simulink model "wheel_dynamics_model"  (R2024b)
settings: Solver=VariableStepAuto  StartTime=0.0  StopTime=3  RelTol=1e-3
undefined symbols (not defined in the file or in its folder): D1, D2, Dm, Dw, gear_ratio, J1, J2, Jm, Js1, Js2, Jw, Ks1, Ks2, tire_loaded_radius
settings Model: VariantFading=off  Creator=bglen  LastModifiedBy=37rst
settings RTWCC: GPUComputeCapability=3.5

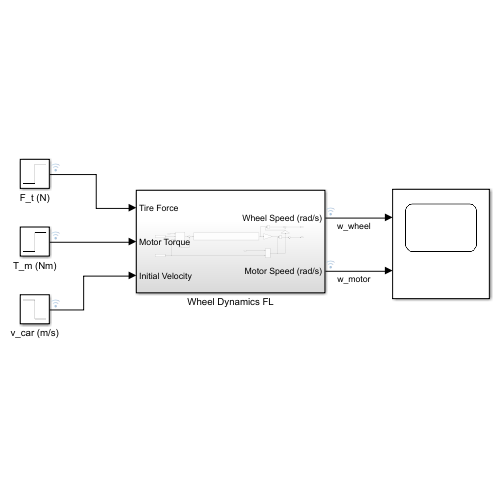
[thumbnail: Simulink's stored preview of the top-level diagram]
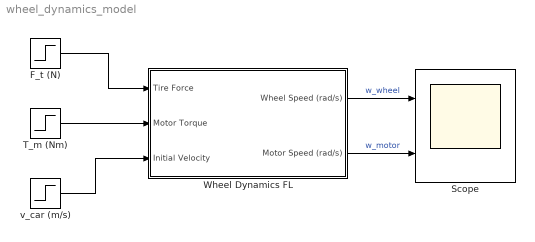
== system wheel_dynamics_model ==
  F_t (N) : Step  Time=2  After=10  SampleTime=0
  Scope : Scope  NumInputPorts=2
  T_m (Nm) : Step  After=5  SampleTime=0
  Wheel Dynamics FL : Subsystem
  v_car (m/s) : Step  Before=1  After=0  SampleTime=0
  wires:
  T_m (Nm)/1 -> Wheel Dynamics FL/2(Motor Torque)
  v_car (m/s)/1 -> Wheel Dynamics FL/3(Initial Velocity)
  F_t (N)/1 -> Wheel Dynamics FL/1(Tire Force)
  Wheel Dynamics FL/1(Wheel Speed (rad/s)) -> Scope/1  "w_wheel"
  Wheel Dynamics FL/2(Motor Speed (rad/s)) -> Scope/2  "w_motor"

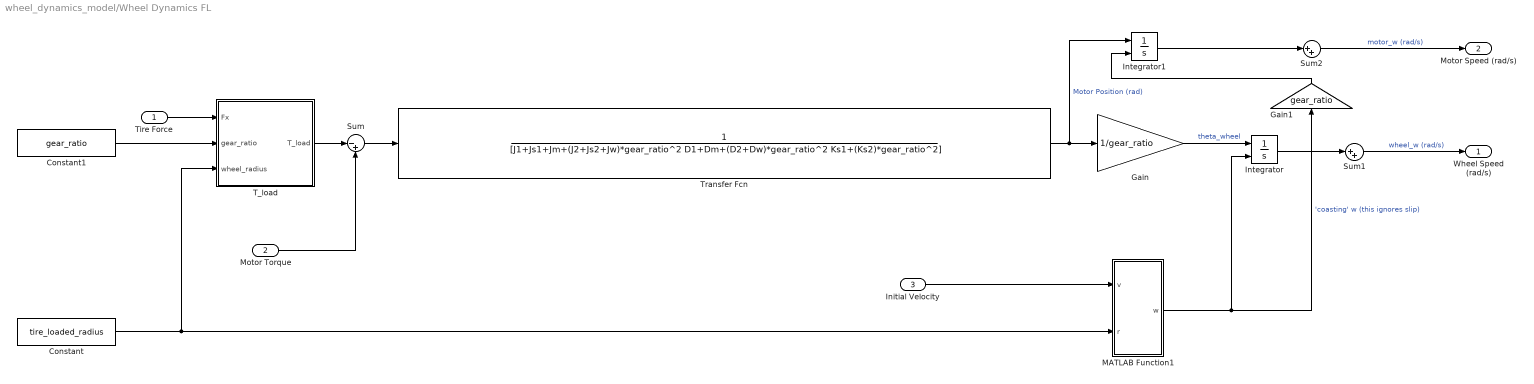
== system wheel_dynamics_model/Wheel Dynamics FL ==
  Tire Force : Inport
  Motor Torque : Inport  Port=2
  Initial Velocity : Inport  Port=3
  Constant : Constant  Value=tire_loaded_radius
  Constant1 : Constant  Value=gear_ratio
  Gain : Gain  Gain=1/gear_ratio
  Gain1 : Gain  Gain=gear_ratio
  Integrator : Integrator  InitialConditionSource=external
  Integrator1 : Integrator  InitialConditionSource=external
  MATLAB Function1 : MATLAB Function  TreatAsAtomicUnit=on
  Sum : Sum  Inputs=|-+
  Sum1 : Sum  Inputs=|++
  Sum2 : Sum  Inputs=|++
  T_load : MATLAB Function  TreatAsAtomicUnit=on
  Transfer Fcn : TransferFcn  Denominator=[J1+Js1+Jm+(J2+Js2+Jw)*gear_ratio^2 D1+Dm+(D2+Dw)*gear_ratio^2 Ks1+(Ks2)*gear_ratio^2]
  Wheel Speed (rad/s) : Outport
  Motor Speed (rad/s) : Outport  Port=2
  wires:
  Motor Torque/1 -> Sum/2
  Tire Force/1 -> T_load/1(Fx)
  T_load/1(T_load) -> Sum/1
  Gain/1 -> Integrator/1  "theta_wheel"
  Initial Velocity/1 -> MATLAB Function1/1(v)
  Constant/1 -> MATLAB Function1/2(r), T_load/3(wheel_radius)
  Sum/1 -> Transfer Fcn/1
  Transfer Fcn/1 -> Integrator1/1, Gain/1  "Motor Position (rad)"
  Integrator/1 -> Sum1/1
  Sum1/1 -> Wheel Speed (rad/s)/1  "wheel_w (rad/s)"
  Constant1/1 -> T_load/2(gear_ratio)
  MATLAB Function1/1(w) -> Gain1/1, Integrator/2  "'coasting' w (this ignores slip)"
  Sum2/1 -> Motor Speed (rad/s)/1  "motor_w (rad/s)"
  Integrator1/1 -> Sum2/1
  Gain1/1 -> Integrator1/2

== matlab function wheel_dynamics_model/Wheel Dynamics FL/MATLAB Function1 ==
  data: v input; w output; r input
function w = fcn(v, r)

w = v/r;

== matlab function wheel_dynamics_model/Wheel Dynamics FL/T_load ==
  data: Fx input; gear_ratio input; T_load output; wheel_radius input
function T_load = fcn(Fx, gear_ratio, wheel_radius)

T_load=wheel_radius*gear_ratio*Fx; % 'load torque' calculation
